simulink model "first2ninth"  (R2018a)
settings: Solver=VariableStepAuto  StartTime=0.0  StopTime=400  RelTol=1e-3
values from neighbouring files (symbols this model uses):
  c = 1.1    [matlab.mat]
  delta = 0.1    [matlab.mat]
  kapa = 37.7189607492    [matlab.mat]
  kd = 0.2    [matlab.mat]
  ki = 0.01    [matlab.mat]
  kp = 0.2    [matlab.mat]
  Qs = 0.125    [matlab.mat]
  R = 1.6    [matlab.mat]
libraries: simulink x1
settings Model: Creator=Master  LastModifiedBy=Master

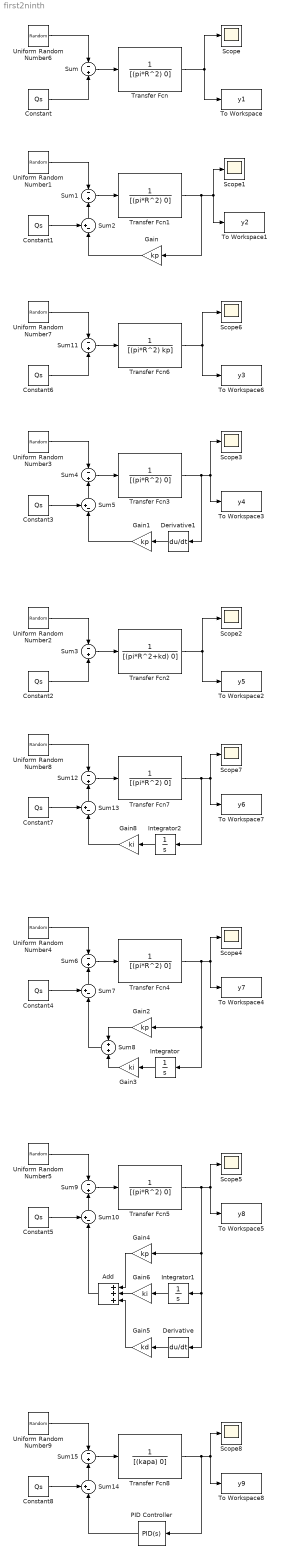
== system first2ninth ==
  Add : Sum  Inputs=+++
  Constant{,1..8} (9 alike) : Constant  Value=Qs
  Derivative : Derivative
  Derivative1 : Derivative
  Gain{,1..2,4} (4 alike) : Gain  Gain=kp
  Gain3 : Gain  Gain=ki
  Gain5 : Gain  Gain=kd
  Gain6 : Gain  Gain=ki
  Gain8 : Gain  Gain=ki
  Integrator : Integrator
  Integrator1 : Integrator
  Integrator2 : Integrator
  PID Controller : simulink/Continuous/PID Controller  Controller=PID  TimeDomain=Continuous-time  SampleTime=-1  IntegratorMethod=Forward Euler  FilterMethod=Forward Euler  Form=Parallel  UseFilter=on  ControllerParametersSource=internal  P=1  I=1  D=0  N=100  InitialConditionSource=internal  InitialConditionForIntegrator=0  InitialConditionForFilter=0  ExternalReset=none  LimitOutput=off  UpperSaturationLimit=inf  LowerSaturationLimit=-inf  LinearizeAsGain=on  AntiWindupMode=none  Kb=1  TrackingMode=off  Kt=1  PParamMin=[]  PParamMax=[]  IParamMin=[]  IParamMax=[]  DParamMin=[]  DParamMax=[]  NParamMin=[]  NParamMax=[]  KbParamMin=[]  KbParamMax=[]  KtParamMin=[]  KtParamMax=[]  POutMin=[]  POutMax=[]  IOutMin=[]  IOutMax=[]  DOutMin=[]  DOutMax=[]  NOutMin=[]  NOutMax=[]  KbOutMin=[]  KbOutMax=[]  KtOutMin=[]  KtOutMax=[]  IntegratorOutMin=[]  IntegratorOutMax=[]  FilterOutMin=[]  FilterOutMax=[]  SumOutMin=[]  SumOutMax=[]  SumI1OutMin=[]  SumI1OutMax=[]  SumI2OutMin=[]  SumI2OutMax=[]  SumI3OutMin=[]  SumI3OutMax=[]  SumDOutMin=[]  SumDOutMax=[]  SaturationOutMin=[]  SaturationOutMax=[]  IntegratorContinuousStateAttributes=''  IntegratorStateMustResolveToSignalObject=off  IntegratorRTWStateStorageClass=Auto  FilterContinuousStateAttributes=''  FilterStateMustResolveToSignalObject=off  FilterRTWStateStorageClass=Auto  DifferentiatorICPrevScaledInput=0  DifferentiatorOutMin=[]  DifferentiatorOutMax=[]  FilterDiffOutCoefMin=[]  FilterDiffOutCoefMax=[]  SumDenOutMin=[]  SumDenOutMax=[]  SumNumOutMin=[]  SumNumOutMax=[]  ReciprocalOutMin=[]  ReciprocalOutMax=[]  DivideOutMin=[]  DivideOutMax=[]  TunerSelectOption=Transfer Function Based (PID Tuner App)
  Scope{,1..8} (9 alike) : Scope
  Sum{,1,3..4,6,9,11..12,15} (9 alike) : Sum  Inputs=-|+
  Sum{2,5,7,10,13..14} (6 alike) : Sum  Inputs=+-|
  Sum8 : Sum  Inputs=+|+
  To Workspace : ToWorkspace  VariableName=y1  SaveFormat=Timeseries  SampleTime=-1
      settings: Save2DSignal=2-D array (concatenate along first dimension)
  To Workspace1 : ToWorkspace  VariableName=y2  SaveFormat=Timeseries  SampleTime=-1
  To Workspace2 : ToWorkspace  VariableName=y5  SaveFormat=Timeseries  SampleTime=-1
  To Workspace3 : ToWorkspace  VariableName=y4  SaveFormat=Timeseries  SampleTime=-1
  To Workspace4 : ToWorkspace  VariableName=y7  SaveFormat=Timeseries  SampleTime=-1
  To Workspace5 : ToWorkspace  VariableName=y8  SaveFormat=Timeseries  SampleTime=-1
  To Workspace6 : ToWorkspace  VariableName=y3  SaveFormat=Timeseries  SampleTime=-1
  To Workspace7 : ToWorkspace  VariableName=y6  SaveFormat=Timeseries  SampleTime=-1
  To Workspace8 : ToWorkspace  VariableName=y9  SaveFormat=Timeseries  SampleTime=-1
  Transfer Fcn{,1,3..5,7} (6 alike) : TransferFcn  Denominator=[(pi*R^2) 0]
  Transfer Fcn2 : TransferFcn  Denominator=[(pi*R^2+kd) 0]
  Transfer Fcn6 : TransferFcn  Denominator=[(pi*R^2) kp]
  Transfer Fcn8 : TransferFcn  Denominator=[(kapa) 0]
  Uniform Random Number{1..9} (9 alike) : UniformRandomNumber  Minimum=(c-delta)*Qs  Maximum=(c+delta)*Qs  SampleTime=0.1
  wires:
  Uniform Random Number6/1 -> Sum/1
  Constant/1 -> Sum/2
  Sum/1 -> Transfer Fcn/1
  Transfer Fcn/1 -> To Workspace/1, Scope/1
  Gain/1 -> Sum2/2
  Uniform Random Number1/1 -> Sum1/1
  Sum2/1 -> Sum1/2
  Sum1/1 -> Transfer Fcn1/1
  Transfer Fcn1/1 -> Gain/1, To Workspace1/1, Scope1/1
  Constant1/1 -> Sum2/1
  Sum3/1 -> Transfer Fcn2/1
  Constant2/1 -> Sum3/2
  Uniform Random Number2/1 -> Sum3/1
  Transfer Fcn2/1 -> To Workspace2/1, Scope2/1
  Constant3/1 -> Sum5/1
  Transfer Fcn3/1 -> Derivative1/1, To Workspace3/1, Scope3/1
  Uniform Random Number3/1 -> Sum4/1
  Sum4/1 -> Transfer Fcn3/1
  Gain1/1 -> Sum5/2
  Sum5/1 -> Sum4/2
  Sum8/1 -> Sum7/2
  Integrator/1 -> Gain3/1
  Uniform Random Number4/1 -> Sum6/1
  Gain3/1 -> Sum8/2
  Gain2/1 -> Sum8/1
  Sum7/1 -> Sum6/2
  Sum6/1 -> Transfer Fcn4/1
  Constant4/1 -> Sum7/1
  Transfer Fcn4/1 -> Integrator/1, Gain2/1, To Workspace4/1, Scope4/1
  Derivative/1 -> Gain5/1
  Add/1 -> Sum10/2
  Gain4/1 -> Add/1
  Sum9/1 -> Transfer Fcn5/1
  Gain5/1 -> Add/3
  Sum10/1 -> Sum9/2
  Uniform Random Number5/1 -> Sum9/1
  Integrator1/1 -> Gain6/1
  Constant5/1 -> Sum10/1
  Transfer Fcn5/1 -> To Workspace5/1, Scope5/1, Derivative/1, Integrator1/1, Gain4/1
  Gain6/1 -> Add/2
  Derivative1/1 -> Gain1/1
  Constant6/1 -> Sum11/2
  Sum11/1 -> Transfer Fcn6/1
  Transfer Fcn6/1 -> To Workspace6/1, Scope6/1
  Uniform Random Number7/1 -> Sum11/1
  Sum13/1 -> Sum12/2
  Constant7/1 -> Sum13/1
  Gain8/1 -> Sum13/2
  Sum12/1 -> Transfer Fcn7/1
  Transfer Fcn7/1 -> Integrator2/1, To Workspace7/1, Scope7/1
  Uniform Random Number8/1 -> Sum12/1
  Integrator2/1 -> Gain8/1
  Sum14/1 -> Sum15/2
  Transfer Fcn8/1 -> PID Controller/1, To Workspace8/1, Scope8/1
  Constant8/1 -> Sum14/1
  Sum15/1 -> Transfer Fcn8/1
  PID Controller/1 -> Sum14/2
  Uniform Random Number9/1 -> Sum15/1
